simulink model "ERGcircobs"  (R2014a)
settings: Solver=ode45  StartTime=0.0  StopTime=25  RelTol=1e-3
libraries: simulink x1
settings Model: Creator=Tigrann  LastModifiedBy=Tigrann

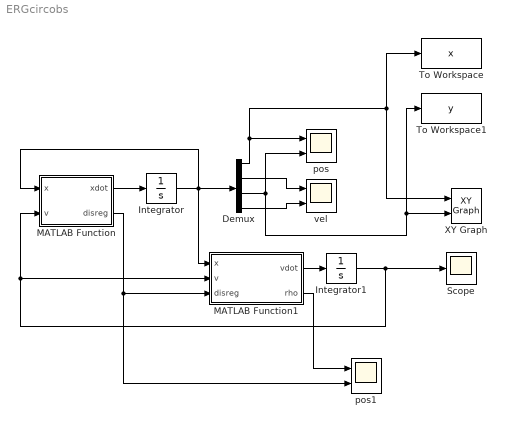
== system ERGcircobs ==
  Demux : Demux
  Integrator : Integrator  InitialCondition=[0.35;0;0.35;0]
  Integrator1 : Integrator  InitialCondition=[0.35;0.35]
  MATLAB Function : MATLAB Function  TreatAsAtomicUnit=on
  MATLAB Function1 : MATLAB Function  TreatAsAtomicUnit=on
  Scope : Scope
      settings: SaveName=v
  To Workspace : ToWorkspace  VariableName=x  SaveFormat=Structure With Time  SampleTime=0.01
  To Workspace1 : ToWorkspace  VariableName=y  SaveFormat=Structure With Time  SampleTime=0.01
  XY Graph : simulink/Sinks/XY Graph  xmin=0  xmax=2  ymin=0  ymax=2  st=-1
  pos : Scope  NumInputPorts=2
      settings: ShowLegends=on  YMin=1.4875~-5  YMax=1.5175~5
  pos1 : Scope  NumInputPorts=2
      settings: ShowLegends=on  YMin=-0.6~0.139948  YMax=1~0.15468
  vel : Scope  NumInputPorts=2
      settings: ShowLegends=on  YMin=-5~-5  YMax=5~5  SaveName=ScopeData2
  wires:
  MATLAB Function/1(xdot) -> Integrator/1
  Integrator/1 -> MATLAB Function/1(x), MATLAB Function1/1(x), Demux/1
  MATLAB Function1/1(vdot) -> Integrator1/1
  Demux/1 -> pos/1, XY Graph/1, To Workspace/1
  Demux/2 -> vel/1
  Demux/3 -> pos/2, To Workspace1/1, XY Graph/2
  Demux/4 -> vel/2
  MATLAB Function1/2(rho) -> pos1/1
  Integrator1/1 -> Scope/1, MATLAB Function1/2(v), MATLAB Function/2(v)
  MATLAB Function/2(disreg) -> MATLAB Function1/3(disreg), pos1/2

== matlab function ERGcircobs/MATLAB Function1 ==
  data: x input; vdot output; v input; rho output; disreg input
function [vdot,rho]= fcn(x,v,disreg)
%#codegen
k=100;
k1=2;
k2=2;
k3=2;
k4=2;
A=[0 1 0 0; -k1 -k2 0 0; 0 0 0 1; 0 0 -k3 -k4];
P=[0.875 -0.5 0 0; -0.5 0.75 0 0; 0  0 0.875 -0.5; 0 0 -0.5 0.75];%lyap(A,Q);
r=[1.8;1.8];

xo1=[1; 0; 0.8; 0]; %obs1 pos
xo2=[1.3; 0; 1.7; 0]; %obs2 pos
d=0.2; %obs rad

deltao1=norm(xo1-[v(1);0;v(2);0])-d-disreg;
deltao2=norm(xo2-[v(1);0;v(2);0])-d-disreg;
delta=min([deltao1 deltao2 (v(1)-disreg) (2-v(1)-disreg) (v(2)-disreg) (2-v(2)-disreg)]);

% deltao1=norm(xo1-x)-d-disreg;
% deltao2=norm(xo2-x)-d-disreg;
% delta=min([deltao1 deltao2 (x(1)-disreg) (2-x(1)-disreg) (x(3)-disreg) (2-x(3)-disreg)]);

%if delta>0
    V=(x-[v(1);0;v(2);0])'*P*(x-[v(1);0;v(2);0]);
    Gamma1=([0;0;-1;0]'*[v(1);0;v(2);0]+0)^2/([0;0;-1;0]'*inv(P)*[0;0;-1;0]);
    Gamma2=([0;0;1;0]'*[v(1);0;v(2);0]-2)^2/([0;0;1;0]'*inv(P)*[0;0;1;0]);
    Gamma3=([-1;0;0;0]'*[v(1);0;v(2);0]+0)^2/([-1;0;0;0]'*inv(P)*[-1;0;0;0]);
    Gamma4=([1;0;0;0]'*[v(1);0;v(2);0]-2)^2/([1;0;0;0]'*inv(P)*[1;0;0;0]);
    xt1=-((xo1-[v(1);0;v(2);0])/(norm(xo1-[v(1);0;v(2);0])))*d+xo1;
    xt2=-((xo2-[v(1);0;v(2);0])/(norm(xo2-[v(1);0;v(2);0])))*d+xo2;
    Gamma5=(2*[(xt1(1)-xo1(1)) 0 (xt1(3)-xo1(3)) 0]*([v(1);0;v(2);0]-xt1))^2/(4*[(xt1(1)-xo1(1)) 0 (xt1(3)-xo1(3)) 0]*inv(P)*[(xt1(1)-xo1(1)) 0 (xt1(3)-xo1(3)) 0]');
    Gamma6=(2*[(xt2(1)-xo2(1)) 0 (xt2(3)-xo2(3)) 0]*([v(1);0;v(2);0]-xt2))^2/(4*[(xt2(1)-xo2(1)) 0 (xt2(3)-xo2(3)) 0]*inv(P)*[(xt2(1)-xo2(1)) 0 (xt2(3)-xo2(3)) 0]');
    Gamma=min([Gamma1 Gamma2 Gamma3 Gamma4 Gamma5 Gamma6]);
    Gamma=max(Gamma,0);
    dis1=sqrt((x(1)-xo1(1))^2+(x(3)-xo1(3))^2);
    dis2=sqrt((x(1)-xo2(1))^2+(x(3)-xo2(3))^2);
    
    paramdelta=0.25; %influence zone of the rep obs
    paramdeltab=0.05;
    
    rho_rep_ob1=max((0.4-dis1+d)/(0.4-paramdelta),0)*[(x(1)-xo1(1))/dis1;(x(3)-xo1(3))/dis1];
    rho_rep_ob2=max((0.4-dis2+d)/(0.4-paramdelta),0)*[(x(1)-xo2(1))/dis2;(x(3)-xo2(3))/dis2];
    rho_rep_b1=max((0.1-([0;0;1;0]'*[x(1);0;x(3);0]+0))/(0.1-paramdeltab),0)*[0;1];
    rho_rep_b2=max((0.1-([0;0;-1;0]'*[x(1);0;x(3);0]+2))/(0.1-paramdeltab),0)*[0;-1];
    rho_rep_b3=max((0.1-([1;0;0;0]'*[x(1);0;x(3);0]+0))/(0.1-paramdeltab),0)*[1;0];
    rho_rep_b4=max((0.1-([-1;0;0;0]'*[x(1);0;x(3);0]+2))/(0.1-paramdeltab),0)*[-1;0];
    rho_at=(r-v)/max(norm(v-r),0.01);
    
    rho=rho_at+rho_rep_ob1+rho_rep_ob2+rho_rep_b1+rho_rep_b2+rho_rep_b3+rho_rep_b4;
    vdot=k*(Gamma-V)*rho;
% else
%     vdot=[0;0];
% end


% plot(x.signals.values,y.signals.values)
% axis([0 2 0 2]);
% hold on
% plot(v.signals.values(:,1), v.signals.values(:,2), 'Color', 'green')
% axis([0 2 0 2]);
% hold on
% xc=[1; 1.3]; %%%depending on xo1 xo2
% yc=[0.5; 1.7]; %%% yo1 yo2
% centers = [xc yc];
% do=0.2; %%% is equal to obs rad
% radii=[do;do];
% viscircles(centers,radii);
% hold on
% Bd=[0 0; 1 0; 0 0; 0 1];
% dx=0.1; %%% depending on disturbance
% dy=0.1; %%% idem
% d=[dx; dy];
% Cpar=1-0.04; %%% safety coeff
% radma=norm(Bd)*norm(d)/Cpar;
% for i=1:100:length(x.signals.values)
%     posact=[v.signals.values(i,1) v.signals.values(i,2)];
%     viscircles(posact,radma,'LineWidth',0.75,'LineStyle','--','EdgeColor','black');
%     hold on
% end

== matlab function ERGcircobs/MATLAB Function ==
  data: x input; xdot output; v input; disreg output
function [xdot,disreg]= fcn(x,v)
%#codegen
k1=2;
k2=2;
k3=2;
k4=2;
A=[0 1 0 0; -k1 -k2 0 0; 0 0 0 1; 0 0 -k3 -k4];% 3rd line 0001 instead of 0010 
B=[0 0;k1 0; 0 0;0 k3];
Bd=[0 0; 1 0; 0 0; 0 1];
dx=0.2;
dy=0.2;
d=[dx; dy];
xdot = A*x+B*v+Bd*d;
Cpar=1-0.04;
disreg=norm(Bd)*norm(d)/Cpar;
